simulink model "vehicle_model_controller"  (R2020b)
settings: Solver=VariableStepAuto  StartTime=0.0  StopTime=10.0  RelTol=1e-3
undefined symbols (not defined in the file or in its folder): BWLF, BWRF, front_forces, FWLF, FWRF, rear_forces
libraries: nesl_utility x24, sdl_lib x16, fl_lib x4, autolibmappedmotor x4, autolibdatasheetbattery x1, vehdynlibsteering x1, pid_lib x1, autolibshared x1
(part 1 of 2)
settings Model: Creator=True  LastModifiedBy=Inver
settings DataIOCC: ExternalInput=half_track_front.getElement(1),[],[],[],[],[],[],[],[],[],[]  LoadExternalInput=on
settings DebuggingCC: ArithmeticOperatorsInVariantConditions=warning
settings SFSimCC: CustomCodeUndefinedFunction=UseInterfaceOnly

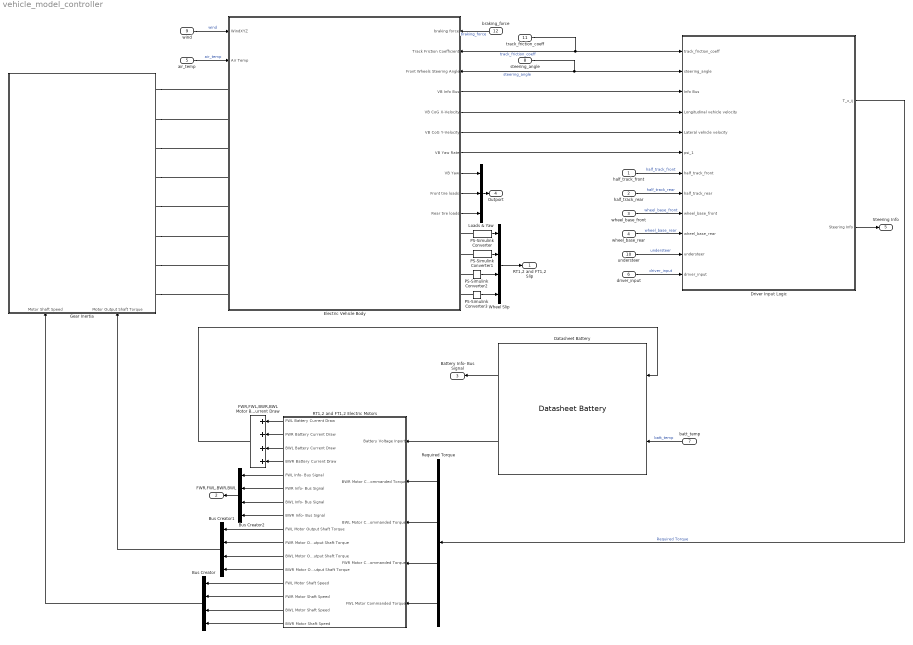
== system vehicle_model_controller ==
  half_track_front : Inport
  half_track_rear : Inport  Port=2
  wheel_base_front : Inport  Port=3
  wheel_base_rear : Inport  Port=4
  air_temp : Inport  Port=5
  driver_input : Inport  Port=6
  batt_temp : Inport  Port=7
  steering_angle : Inport  Port=8
  wind : Inport  Port=9
  understeer : Inport  Port=10
  track_friction_coeff : Inport  Port=11
  braking_force : Inport  Port=12
  Bus Creator : BusCreator  Inputs=FWL Speed,FWR Speed,BWL Speed,BWR Speed
  Bus Creator1 : BusCreator  Inputs=FWL Torque,FWR Torque,BWL Torque,BWR Torque
  Bus Creator2 : BusCreator  Inputs=4
  Datasheet Battery : autolibdatasheetbattery/Datasheet Battery  CapacityCtrl=Parameter  OutputVlt=Unfiltered  BattChargeMax=100  Em=[2.8 3.228 3.284 3.361 3.408 3.427 3.472 3.477 3.493 3.504 3.516 3.528 3.537 3.545 3.555 3.561 3.566 3.576 3.587 3.589 3.594 3.6 3.608 3.61 3.616 3.619 3.626 3.632 3.637 3.64 3.645 3.646 3.652 3.655 3.658 3.661 3.664 3.668 3.673 3.678 3.68 3.681 3.686 3.692 3.699 3.702 3.705 3.71 3.717 3.723 3.728 3.733 3.735 3.742 3.749 3.755 3.761 3.768 3.773 3.78 3.791 3.798 3.798 3.814 3.818 3.825 3.841 3.846 3.855 3.863 3.877 3.885 3.894 3.907 3.919 3.926 3.935 3.944 3.954 3.964 3.974 3.988 3.998 4.014 4.029 4.034 4.047 4.065 4.074 4.086 4.097 4.131 4.126 4.138 4.15 4.18 4.174 4.187 4.207 4.231 4.221]  CapLUTBp=[0 0.01 0.02 0.03 0.04 0.05 0.06 0.07 0.08 0.09 0.1 0.11 0.12 0.13 0.14 0.15 0.16 0.17 0.18 0.19 0.2 0.21 0.22 0.23 0.24 0.25 0.26 0.27 0.28 0.29 0.3 0.31 0.32 0.33 0.34 0.35 0.36 0.37 0.38 0.39 0.4 0.41 0.42 0.43 0.44 0.45 0.46 0.47 0.48 0.49 0.5 0.51 0.52 0.53 0.54 0.55 0.56 0.57 0.58 0.59 0.6 0.61 0.62 0.63 0.64 0.65 0.66 0.67 0.68 0.69 0.7 0.71 0.72 0.73 0.74 0.75 0.76 0.77 0.78 0.79 0.8 0.81 0.82 0.83 0.84 0.85 0.86 0.87 0.88 0.89 0.9 0.91 0.92 0.93 0.94 0.95 0.96 0.97 0.98 0.99 1]  RInt=[0.008846 0.009319 0.009027 0.00847 0.01032 0.01314;0.006389 0.006554 0.005553 0.005525 0.006043 0.007805;0.004364 0.004101 0.00406 0.003452 0.003846 0.004517;0.002031 0.002563 0.002532 0.00246 0.002716 0.003047;0.001443 0.001825 0.001795 0.001778 0.001924 0.002234;0.0005603 0.0007192 0.0006887 0.0007557 0.0007355 0.001014;0.001028 0.001338 0.001 0.001536 0.001546 0.002789]  BattTempBp=[243.1 253.1 263.1 273.1 283.1 298.1 313.1]  CapSOCBp=[0 0.2 0.4 0.6 0.8 1]  Ns=1  Np=1  BattCapInit=100  Tc=1/1000  Vinit=4.221  RefBlkName='autolibdatasheetbattery/Datasheet Battery'
      settings: SourceProductBaseCode=PW
  Driver Input Logic : Subsystem
  Electric Vehicle Body : Subsystem
      settings: PortSchema="{\"entries\":[{\"content\":{\"sides\":[{\"content\":{\"connectorIds\":[\"In1\",\"In2\",\"LConn1\",\"LConn2\",\"LConn3\",\"LConn4\",\"LConn5\",\"LConn6\",\"LConn7\",\"LConn8\"]},\"type\":\"ConnectorPlacement.EquallySpacedRectSide\",\"uuid\":\"d116468d-7868-487f-a964-21d40fbcc809\"},{\"content\":{\"connectorIds\":[\"In3\",\"In4\",\"In5\",\"Out1\",\"Out2\",\"Out3\",\"Out4\",\"Out5\",\"Out6\",\"Out7\",\"RConn1\",\"RConn2\",\"RConn3\",\"RConn4\"],\"side\":\"RIGHT\"},\"type\":\"ConnectorPlacement.EquallySpacedRectSide\",\"uuid\":\"69901164-3ba1-4787-94a1-b6dad3f5570f\"},{\"content\":{\"connectorIds\":[],\"side\":\"TOP\"},\"type\":\"ConnectorPlacement.EquallySpacedRectSide\",\"uuid\":\"0399aa14-7cbc-406a-a0bc-5234930aa618\"},{\"content\":{\"connectorIds\":[],\"side\":\"HIDDEN\"},\"type\":\"ConnectorPlacement.EquallySpacedRectSide\",\"uuid\":\"c7425876-ea80-44ac-a5c9-676a45313985\"}]},\"type\":\"ConnectorPlacement.EquallySpacedConnector\",\"uuid\":\"33585625-d9f5-41d4-8b4d-b29cb62e09b6\"}],\"packageUris\":[\"http://schema.mathworks.com/mf0/Connector/R2020b\"],\"version\":\"1.0\"}"
  FWR,FWL,BWR,BWL Motor Battery Current Draw : Sum  Inputs=++++
  Gear Inertia : Subsystem
      settings: PortSchema="{\"entries\":[{\"content\":{\"sides\":[{\"content\":{\"connectorIds\":[]},\"type\":\"ConnectorPlacement.EquallySpacedRectSide\",\"uuid\":\"d2da853d-f72f-405f-97f5-14de81bcd5cf\"},{\"content\":{\"connectorIds\":[\"RConn1\",\"RConn2\",\"RConn3\",\"RConn4\",\"RConn5\",\"RConn6\",\"RConn7\",\"RConn8\"],\"side\":\"RIGHT\"},\"type\":\"ConnectorPlacement.EquallySpacedRectSide\",\"uuid\":\"46df577e-3ff5-4d09-9a0c-c2313587257d\"},{\"content\":{\"connectorIds\":[],\"side\":\"TOP\"},\"type\":\"ConnectorPlacement.EquallySpacedRectSide\",\"uuid\":\"3ac7701d-a0be-47f8-b1ff-78174d996b09\"},{\"content\":{\"connectorIds\":[\"In1\",\"In2\"],\"side\":\"BOTTOM\"},\"type\":\"ConnectorPlacement.EquallySpacedRectSide\",\"uuid\":\"cde220f9-0c3d-4970-b228-0d476a2943e7\"},{\"content\":{\"connectorIds\":[],\"side\":\"HIDDEN\"},\"type\":\"ConnectorPlacement.EquallySpacedRectSide\",\"uuid\":\"76366aef-65a3-435b-b679-82e74c90300f\"}]},\"type\":\"ConnectorPlacement.EquallySpacedConnector\",\"uuid\":\"e97a27ad-84e2-4fc1-b928-f989677c188c\"}],\"packageUris\":[\"http://schema.mathworks.com/mf0/Connector/R2020b\"],\"version\":\"1.0\"}"
  Loads & Yaw : Mux  Inputs=3
  PS-Simulink Converter{,1..3} (4 alike) : nesl_utility/PS-Simulink Converter  PhysicalDomain=network_engine_domain  SubClassName=ps_output  LeftPortType=input  RightPortType=output  PseudoPeriodic=off  Frequencies=[]  Unit=inherit  AffineConversion=off
  RT1,2 and FT1,2 Electric Motors : Subsystem
  Required Torque : Demux
  Wheel Slip : Mux
  RT1,2 and FT1,2 Slip : Outport
  FWR,FWL,BWR,BWL : Outport  Port=2
  Battery Info- Bus Signal : Outport  Port=3
  Outport : Outport  Port=4
  Steering Info : Outport  Port=5
  wires:
  Datasheet Battery/2 -> RT1,2 and FT1,2 Electric Motors/1(Battery Voltage Inport)
  RT1,2 and FT1,2 Electric Motors/1(FWL Battery Current Draw) -> FWR,FWL,BWR,BWL Motor Battery Current Draw/1
  RT1,2 and FT1,2 Electric Motors/2(FWR Battery Current Draw) -> FWR,FWL,BWR,BWL Motor Battery Current Draw/2
  RT1,2 and FT1,2 Electric Motors/3(BWL Battery Current Draw) -> FWR,FWL,BWR,BWL Motor Battery Current Draw/3
  RT1,2 and FT1,2 Electric Motors/4(BWR Battery Current Draw) -> FWR,FWL,BWR,BWL Motor Battery Current Draw/4
  FWR,FWL,BWR,BWL Motor Battery Current Draw/1 -> Datasheet Battery/1
  PS-Simulink Converter/1 -> Wheel Slip/1
  PS-Simulink Converter1/1 -> Wheel Slip/2
  PS-Simulink Converter2/1 -> Wheel Slip/3
  PS-Simulink Converter3/1 -> Wheel Slip/4
  Wheel Slip/1 -> RT1,2 and FT1,2 Slip/1
  RT1,2 and FT1,2 Electric Motors/5(FWL Info- Bus Signal) -> Bus Creator2/1
  RT1,2 and FT1,2 Electric Motors/6(FWR Info- Bus Signal) -> Bus Creator2/2
  RT1,2 and FT1,2 Electric Motors/7(BWL Info- Bus Signal) -> Bus Creator2/3
  RT1,2 and FT1,2 Electric Motors/8(BWR Info- Bus Signal) -> Bus Creator2/4
  RT1,2 and FT1,2 Electric Motors/14(FWR Motor Shaft Speed) -> Bus Creator/2
  RT1,2 and FT1,2 Electric Motors/15(BWL Motor Shaft Speed) -> Bus Creator/3
  RT1,2 and FT1,2 Electric Motors/16(BWR Motor Shaft Speed) -> Bus Creator/4
  RT1,2 and FT1,2 Electric Motors/13(FWL Motor Shaft Speed) -> Bus Creator/1
  Datasheet Battery/1 -> Battery Info- Bus Signal/1
  RT1,2 and FT1,2 Electric Motors/9(FWL Motor Output Shaft Torque) -> Bus Creator1/1
  RT1,2 and FT1,2 Electric Motors/10(FWR Motor Output Shaft Torque) -> Bus Creator1/2
  RT1,2 and FT1,2 Electric Motors/11(BWL Motor Output Shaft Torque) -> Bus Creator1/3
  RT1,2 and FT1,2 Electric Motors/12(BWR Motor Output Shaft Torque) -> Bus Creator1/4
  Required Torque/4 -> RT1,2 and FT1,2 Electric Motors/5(FWL Motor Commanded Torque)
  Required Torque/3 -> RT1,2 and FT1,2 Electric Motors/4("FWR Motor Commanded Torque ")
  Required Torque/2 -> RT1,2 and FT1,2 Electric Motors/3(BWL Motor Commanded Torque)
  Required Torque/1 -> RT1,2 and FT1,2 Electric Motors/2(BWR Motor Commanded Torque)
  Loads & Yaw/1 -> Outport/1
  Electric Vehicle Body/5(VB Yaw) -> Loads & Yaw/1
  Electric Vehicle Body/6(Front tire loads) -> Loads & Yaw/2
  Electric Vehicle Body/7(Rear tire loads) -> Loads & Yaw/3
  Bus Creator2/1 -> FWR,FWL,BWR,BWL/1
  Bus Creator1/1 -> Gear Inertia/2(Motor Output Shaft Torque)
  Bus Creator/1 -> Gear Inertia/1(Motor Shaft Speed)
  air_temp/1 -> Electric Vehicle Body/2(Air Temp)  "air_temp"
  wind/1 -> Electric Vehicle Body/1(WindXYZ)  "wind"
  batt_temp/1 -> Datasheet Battery/2  "batt_temp"
  track_friction_coeff/1 -> Driver Input Logic/1(track_friction_coeff), Electric Vehicle Body/4(Track Friction Coefficient)  "track_friction_coeff"
  steering_angle/1 -> Electric Vehicle Body/5(Front Wheels Steering Angle), Driver Input Logic/2(steering_angle)  "steering_angle"
  Electric Vehicle Body/1(VB Info Bus) -> Driver Input Logic/3(Info Bus)
  Electric Vehicle Body/2("VB CoG X-Velocity ") -> Driver Input Logic/4(Longitudinal vehicle velocity)
  Electric Vehicle Body/3(VB CoG Y-Velocity) -> Driver Input Logic/5(Lateral vehicle velocity)
  Electric Vehicle Body/4(VB Yaw Rate) -> Driver Input Logic/6(psi_1)
  half_track_front/1 -> Driver Input Logic/7(half_track_front)  "half_track_front"
  half_track_rear/1 -> Driver Input Logic/8(half_track_rear)  "half_track_rear"
  wheel_base_front/1 -> Driver Input Logic/9(wheel_base_front)  "wheel_base_front"
  wheel_base_rear/1 -> Driver Input Logic/10(wheel_base_rear)  "wheel_base_rear"
  understeer/1 -> Driver Input Logic/11(understeer)  "understeer"
  driver_input/1 -> Driver Input Logic/12(driver_input)  "driver_input"
  Driver Input Logic/1(T_x_ij) -> Required Torque/1  "Required Torque"
  Driver Input Logic/2(Steering Info) -> Steering Info/1
  braking_force/1 -> Electric Vehicle Body/3(braking force)  "braking_force"
  connections:
  PS-Simulink Converter/LConn1 -- Electric Vehicle Body/RConn1
  PS-Simulink Converter1/LConn1 -- Electric Vehicle Body/RConn2
  PS-Simulink Converter2/LConn1 -- Electric Vehicle Body/RConn3
  PS-Simulink Converter3/LConn1 -- Electric Vehicle Body/RConn4
  Gear Inertia/RConn1 -- Electric Vehicle Body/LConn1
  Gear Inertia/RConn2 -- Electric Vehicle Body/LConn2
  Gear Inertia/RConn3 -- Electric Vehicle Body/LConn3
  Gear Inertia/RConn4 -- Electric Vehicle Body/LConn4
  Gear Inertia/RConn5 -- Electric Vehicle Body/LConn5
  Gear Inertia/RConn6 -- Electric Vehicle Body/LConn6
  Gear Inertia/RConn7 -- Electric Vehicle Body/LConn7
  Gear Inertia/RConn8 -- Electric Vehicle Body/LConn8

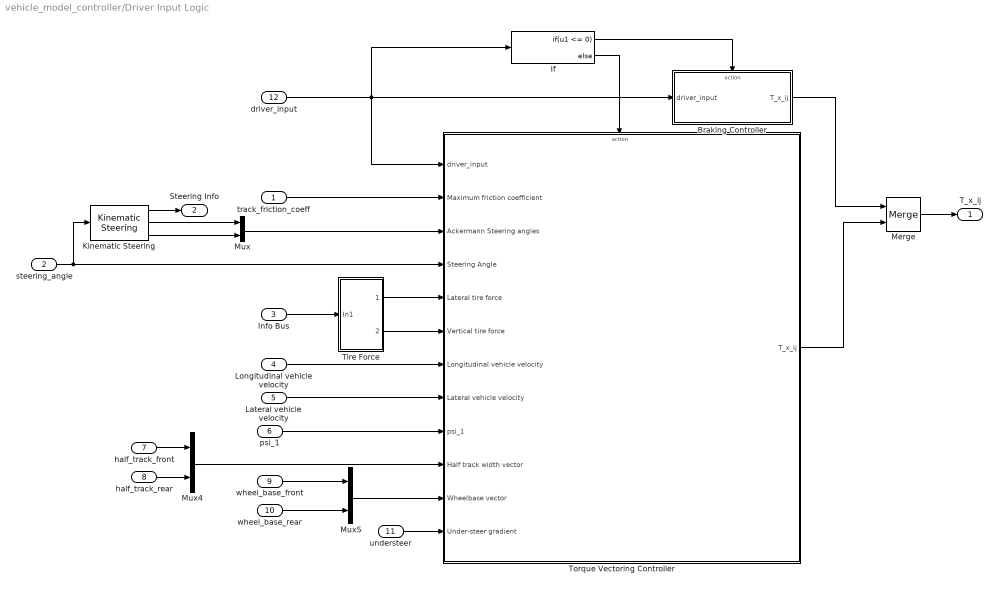
== system vehicle_model_controller/Driver Input Logic ==
  track_friction_coeff : Inport
  steering_angle : Inport  Port=2
  Info Bus : Inport  Port=3
  Longitudinal vehicle velocity : Inport  Port=4
  Lateral vehicle velocity : Inport  Port=5
  psi_1 : Inport  Port=6
  half_track_front : Inport  Port=7
  half_track_rear : Inport  Port=8
  wheel_base_front : Inport  Port=9
  wheel_base_rear : Inport  Port=10
  understeer : Inport  Port=11
  driver_input : Inport  Port=12
  Braking Controller : Subsystem
  If : If  IfExpression=u1 <= 0
  Kinematic Steering : vehdynlibsteering/Kinematic Steering  StrgType=Ackerman  StrgRatioType=Constant  Loc=Front  NrmlFctr=0.01  TrckWdth=1  WhlBase=1.524  Db=0  StrgRng=1.25*pi  StrgAngBpts="[-6.2832   -5.0265   -3.7699   -2.5133   -1.2566         0    1.2566    2.5133    3.7699    5.0265    6.2832]"  StrgRatioTbl=|  StrgRatio=100  StrgArmLngth=0.1  RckCsLngth=0.5  TieRodLngth=0.248  D=0.2  PnnRadius=0.0057  PnnRadiusTbl="[0.0055    0.0055    0.0056    0.0057    0.0058    0.0057    0.0057    0.0057    0.0056    0.0055    0.0055]"  RodLngth=0.1  ParaArmLngth=0.9  aMode=2
      | [13.5000   13.3750   13.2500   13.1250   13.0000   13.0000   13.0000   13.1250   13.2500   13.3750   13.5000
      | ]
  Merge : Merge
  Mux : Mux  Inputs=2
  Mux4 : Mux  Inputs=2
  Mux5 : Mux  Inputs=2
  Tire Force : Subsystem
  Torque Vectoring Controller : Subsystem
  T_x_ij : Outport
  Steering Info : Outport  Port=2
  wires:
  Mux4/1 -> Torque Vectoring Controller/10(Half track width vector)
  understeer/1 -> Torque Vectoring Controller/12(Under-steer gradient)
  Tire Force/1(Lateral) -> Torque Vectoring Controller/5(Lateral tire force)
  Lateral vehicle velocity/1 -> Torque Vectoring Controller/8(Lateral vehicle velocity)
  Mux5/1 -> Torque Vectoring Controller/11(Wheelbase vector)
  Longitudinal vehicle velocity/1 -> Torque Vectoring Controller/7(Longitudinal vehicle velocity)
  Tire Force/2(Vertical) -> Torque Vectoring Controller/6(Vertical tire force)
  Info Bus/1 -> Tire Force/1(In1)
  half_track_front/1 -> Mux4/1
  half_track_rear/1 -> Mux4/2
  wheel_base_rear/1 -> Mux5/2
  wheel_base_front/1 -> Mux5/1
  psi_1/1 -> Torque Vectoring Controller/9(psi_1)
  track_friction_coeff/1 -> Torque Vectoring Controller/2(Maximum friction coefficient)
  If/1 -> Braking Controller/Action
  Merge/1 -> T_x_ij/1
  If/2 -> Torque Vectoring Controller/Action
  Braking Controller/1(T_x_ij) -> Merge/1
  Torque Vectoring Controller/1(T_x_ij) -> Merge/2
  driver_input/1 -> Braking Controller/1(driver_input), Torque Vectoring Controller/1(driver_input), If/1
  Kinematic Steering/3 -> Mux/2
  Kinematic Steering/2 -> Mux/1
  steering_angle/1 -> Torque Vectoring Controller/4(Steering Angle), Kinematic Steering/1
  Mux/1 -> Torque Vectoring Controller/3("Ackermann Steering angles ")
  Kinematic Steering/1 -> Steering Info/1

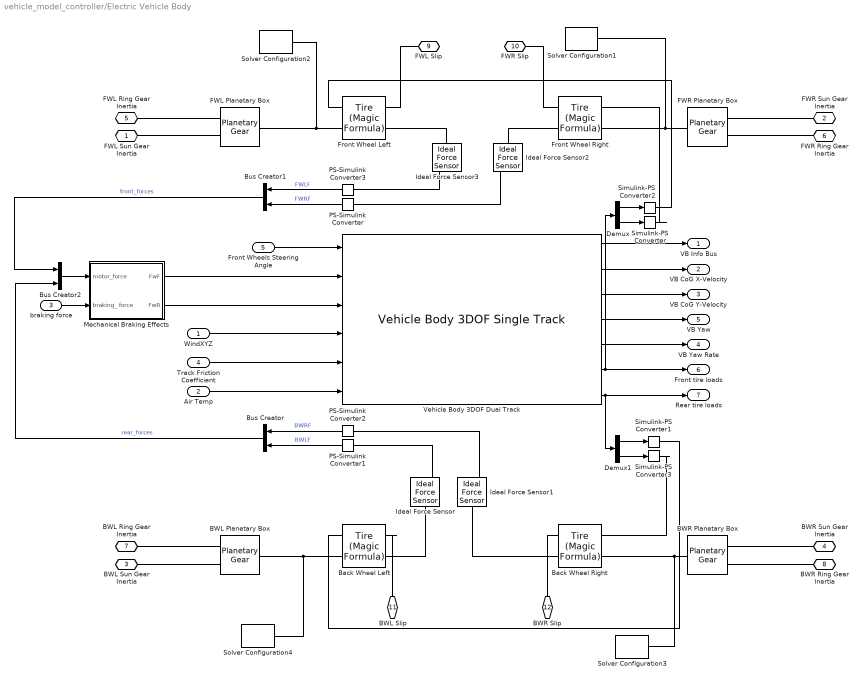
== system vehicle_model_controller/Electric Vehicle Body ==
  WindXYZ : Inport
  Air Temp : Inport  Port=2
  braking force : Inport  Port=3
  Track Friction Coefficient : Inport  Port=4
  Front Wheels Steering Angle : Inport  Port=5
  BWL Planetary Box : sdl_lib/Gears/Planetary Gear  rs_ratio=2  friction_model=sdl.enum.gear_friction.none  mu_visc=[0, 0] N*m/(rad/s)  efficiency=[.96, .98]  temperature_TLU=[280, 300, 320] K  efficiency_sp_TLU=[.95, .9, .85]  efficiency_rp_TLU=[.95, .9, .85]  pwr_thr=[.001, .001] W  thermal_mass=50 J/K  T_init=300 K  model_inertia=simscape.enum.onoff.off  planet_inertia=0.001 kg*m^2
      settings: SourceProductBaseCode=LD
  BWR Planetary Box : sdl_lib/Gears/Planetary Gear  rs_ratio=2  friction_model=sdl.enum.gear_friction.none  mu_visc=[0, 0] N*m/(rad/s)  efficiency=[.96, .98]  temperature_TLU=[280, 300, 320] K  efficiency_sp_TLU=[.95, .9, .85]  efficiency_rp_TLU=[.95, .9, .85]  pwr_thr=[.001, .001] W  thermal_mass=50 J/K  T_init=300 K  model_inertia=simscape.enum.onoff.off  planet_inertia=0.001 kg*m^2
      settings: SourceProductBaseCode=LD
  Back Wheel Left : sdl_lib/Tires & Vehicles/Tire (Magic Formula)  parameterization=sdl.enum.magic_tire_model.peak  F_z1=3000 N  F_x1=3500 N  kappa1=10  B_m=10  C_m=1.9  D_m=1  E_m=0.97  fz0=4000 N  p_Cx=1.685  p_Dx=[1.21, -.037]  p_Ex=[.344, .095, -.02, 0]  p_Kx=[21.51, -.163, .245]  p_Hx=[-.002, .002]  p_Vx=[0, 0]  v_tr_thr=0.1 m/s  r_e=0.3 m  model_compliance=0  stiffness=1e6 N/m  damping=1000 N/(m/s)  model_inertia=0  inertia=1 kg*m^2  initial_velocity=0 rad/s  model_resistance=0  resistance_model=1  coeff=0.015  p_tire=250e3 Pa  alpha=-0.003  beta=0.97  coeff_a=84e-4  coeff_b=6.2e-4 s/m  coeff_c=1.6e-4 s^2/m^2  v_thr=0.001 m/s
  Back Wheel Right : sdl_lib/Tires & Vehicles/Tire (Magic Formula)  parameterization=sdl.enum.magic_tire_model.peak  F_z1=3000 N  F_x1=3500 N  kappa1=10  B_m=10  C_m=1.9  D_m=1  E_m=0.97  fz0=4000 N  p_Cx=1.685  p_Dx=[1.21, -.037]  p_Ex=[.344, .095, -.02, 0]  p_Kx=[21.51, -.163, .245]  p_Hx=[-.002, .002]  p_Vx=[0, 0]  v_tr_thr=0.1 m/s  r_e=0.3 m  model_compliance=0  stiffness=1e6 N/m  damping=1000 N/(m/s)  model_inertia=0  inertia=1 kg*m^2  initial_velocity=0 rad/s  model_resistance=0  resistance_model=1  coeff=0.015  p_tire=250e3 Pa  alpha=-0.003  beta=0.97  coeff_a=84e-4  coeff_b=6.2e-4 s/m  coeff_c=1.6e-4 s^2/m^2  v_thr=0.001 m/s
  Bus Creator : BusCreator  Inputs=BWRF,BWLF
  Bus Creator1 : BusCreator  Inputs=FWLF,FWRF
  Bus Creator2 : BusCreator  Inputs=front_forces,rear_forces
  Demux : Demux  Outputs=2
  Demux1 : Demux  Outputs=2
  FWL Planetary Box : sdl_lib/Gears/Planetary Gear  rs_ratio=2  friction_model=sdl.enum.gear_friction.none  mu_visc=[0, 0] N*m/(rad/s)  efficiency=[.96, .98]  temperature_TLU=[280, 300, 320] K  efficiency_sp_TLU=[.95, .9, .85]  efficiency_rp_TLU=[.95, .9, .85]  pwr_thr=[.001, .001] W  thermal_mass=50 J/K  T_init=300 K  model_inertia=simscape.enum.onoff.off  planet_inertia=0.001 kg*m^2
      settings: SourceProductBaseCode=LD
  FWR Planetary Box : sdl_lib/Gears/Planetary Gear  rs_ratio=2  friction_model=sdl.enum.gear_friction.none  mu_visc=[0, 0] N*m/(rad/s)  efficiency=[.96, .98]  temperature_TLU=[280, 300, 320] K  efficiency_sp_TLU=[.95, .9, .85]  efficiency_rp_TLU=[.95, .9, .85]  pwr_thr=[.001, .001] W  thermal_mass=50 J/K  T_init=300 K  model_inertia=simscape.enum.onoff.off  planet_inertia=0.001 kg*m^2
      settings: SourceProductBaseCode=LD
  Front Wheel Left : sdl_lib/Tires & Vehicles/Tire (Magic Formula)  parameterization=sdl.enum.magic_tire_model.peak  F_z1=3000 N  F_x1=3500 N  kappa1=10  B_m=10  C_m=1.9  D_m=1  E_m=0.97  fz0=4000 N  p_Cx=1.685  p_Dx=[1.21, -.037]  p_Ex=[.344, .095, -.02, 0]  p_Kx=[21.51, -.163, .245]  p_Hx=[-.002, .002]  p_Vx=[0, 0]  v_tr_thr=0.1 m/s  r_e=0.3 m  model_compliance=0  stiffness=1e6 N/m  damping=1000 N/(m/s)  model_inertia=0  inertia=1 kg*m^2  initial_velocity=0 rad/s  model_resistance=0  resistance_model=1  coeff=0.015  p_tire=250e3 Pa  alpha=-0.003  beta=0.97  coeff_a=84e-4  coeff_b=6.2e-4 s/m  coeff_c=1.6e-4 s^2/m^2  v_thr=0.001 m/s
  Front Wheel Right : sdl_lib/Tires & Vehicles/Tire (Magic Formula)  parameterization=sdl.enum.magic_tire_model.peak  F_z1=3000 N  F_x1=3500 N  kappa1=10  B_m=10  C_m=1.9  D_m=1  E_m=0.97  fz0=4000 N  p_Cx=1.685  p_Dx=[1.21, -.037]  p_Ex=[.344, .095, -.02, 0]  p_Kx=[21.51, -.163, .245]  p_Hx=[-.002, .002]  p_Vx=[0, 0]  v_tr_thr=0.1 m/s  r_e=0.3 m  model_compliance=0  stiffness=1e6 N/m  damping=1000 N/(m/s)  model_inertia=0  inertia=1 kg*m^2  initial_velocity=0 rad/s  model_resistance=0  resistance_model=1  coeff=0.015  p_tire=250e3 Pa  alpha=-0.003  beta=0.97  coeff_a=84e-4  coeff_b=6.2e-4 s/m  coeff_c=1.6e-4 s^2/m^2  v_thr=0.001 m/s
  Ideal Force Sensor{,1..3} (4 alike) : fl_lib/Mechanical/Mechanical Sensors/Ideal Force Sensor
  Mechanical Braking Effects : Subsystem
  PS-Simulink Converter{,1..3} (4 alike) : nesl_utility/PS-Simulink Converter  PhysicalDomain=network_engine_domain  SubClassName=ps_output  LeftPortType=input  RightPortType=output  PseudoPeriodic=off  Frequencies=[]  Unit=inherit  AffineConversion=off
  Simulink-PS Converter{,1..3} (4 alike) : nesl_utility/Simulink-PS Converter  PhysicalDomain=network_engine_domain  SubClassName=ps_input  LeftPortType=input  RightPortType=output  PseudoPeriodic=off  Frequencies=[]  NoiseDistribution=none  NoiseParameters=[]  Unit=N  AffineConversion=off  FilteringAndDerivatives=provide  SimscapeFilterOrder=1  InputFilterTimeConstant=0.001  UdotUserProvided=0
  Solver Configuration{1..4} (4 alike) : nesl_utility/Solver Configuration  PhysicalDomain=network_engine_domain  SubClassName=solver  LeftPortType=input  RightPortType=generic  Tones=[]  Harmonics=[]  SimulateNoise=off  Profile=off  UseLocalSampling=off  EnableSwitchedLinearOptims=on  FrequencyDomain=off  UseCCode=off  RelTol=0.001  AbsTol=1e-06  MinStep=1e-09  ToWorkspace=off  RevertToSquareIcSolve=off  NumHomotopyIterations=100  PhasorMode=off  PhasorModeNumHarmonics=1  DoDC=off  ResidualTolerance=1e-09  UseLocalSolver=off  LocalSolverChoice=NE_BACKWARD_EULER_ADVANCER  LocalSolverSampleTime=0.001  DoFixedCost=off  MaxNonlinIter=3  MaxModeIter=2  ComputeImpulses=off  ImpulseIterations=2  LinearAlgebra=auto  EquationFormulation=NE_TIME_EF  DelaysMemoryBudget=1024  AutomaticFiltering=on  FilteringTimeConstant=0.001  PartitionStorageMethod=AS_NEEDED  PartitionMemoryBudget=1024  PartitionMethod=ROBUST
  Vehicle Body 3DOF Dual Track : autolibshared/Vehicle Body 3DOF Single Track  trackMode=Dual  inputMode=External longitudinal forces  frontSteerMode=on  rearSteerMode=off  windMode=on  muMode=on  extFMode=off  extMMode=off  htchFMode=off  htchMMode=off  extXo=off  extpsio=off  extxdoto=off  extro=off  extYo=off  extTamb=on  extydoto=off  aMode=2  NF=2  NR=2  m=223  a=1.5  b=1.5  h=0.35  dh=1  hh=0.2  X_o=0  xdot_o=0  CalphaMode=off  sigmaMode=on  d=0  hl=0  w=[1.4,1.4]  Cy_f=12e3  Cy_r=11e3  sigma_f=.1  sigma_r=.1  alpha_f_brk=[-.1 .1]  Cy_f_data=[-9e3 9e3]  alpha_r_brk=[-.1 .1]  Cy_r_data=[-9e3 9e3]  Y_o=0  ydot_o=0  Izz=4000  psi_o=0  r_o=0  Af=2  Cd=.3  Cl=.1  Cpm=.1  beta_w=[0:0.01:0.3]  Cs=[0:0.03:0.9]  Cym=[0:0.01:0.3]  Pabs=101325  Tair=273  g=9.81  mu=1  xdot_tol=.01  Fznom=5000  Fxtire_sat=7e4  Fytire_sat=7e4  longOff=0  latOff=0  vertOff=0  wrapAng=off
      settings: SourceProductBaseCode=PW,MT,UV,VE,VP
  FWL Sun Gear Inertia : PMIOPort  Side=Left
  FWR Sun Gear Inertia : PMIOPort  Port=2  Side=Left
  BWL Sun Gear Inertia : PMIOPort  Port=3  Side=Left
  BWR Sun Gear Inertia : PMIOPort  Port=4  Side=Left
  FWL Ring Gear Inertia : PMIOPort  Port=5  Side=Left
  FWR Ring Gear Inertia : PMIOPort  Port=6  Side=Left
  BWL Ring Gear Inertia : PMIOPort  Port=7  Side=Left
  BWR Ring Gear Inertia : PMIOPort  Port=8  Side=Left
  FWL Slip : PMIOPort  Port=9  Side=Right
  FWR Slip : PMIOPort  Port=10  Side=Right
  BWL Slip : PMIOPort  Port=11  Side=Right
  BWR Slip : PMIOPort  Port=12  Side=Right
  VB Info Bus : Outport
  "VB CoG X-Velocity " : Outport  Port=2
  VB CoG Y-Velocity : Outport  Port=3
  VB Yaw Rate : Outport  Port=4
  VB Yaw : Outport  Port=5
  Front tire loads : Outport  Port=6
  Rear tire loads : Outport  Port=7
  wires:
  Vehicle Body 3DOF Dual Track/6 -> Front tire loads/1, Demux/1
  Vehicle Body 3DOF Dual Track/7 -> Rear tire loads/1, Demux1/1
  Air Temp/1 -> Vehicle Body 3DOF Dual Track/6
  Front Wheels Steering Angle/1 -> Vehicle Body 3DOF Dual Track/1
  Track Friction Coefficient/1 -> Vehicle Body 3DOF Dual Track/5
  WindXYZ/1 -> Vehicle Body 3DOF Dual Track/4
  Vehicle Body 3DOF Dual Track/1 -> VB Info Bus/1
  Vehicle Body 3DOF Dual Track/2 -> "VB CoG X-Velocity "/1
  Vehicle Body 3DOF Dual Track/3 -> VB CoG Y-Velocity/1
  Vehicle Body 3DOF Dual Track/4 -> VB Yaw/1
  Vehicle Body 3DOF Dual Track/5 -> VB Yaw Rate/1
  Mechanical Braking Effects/2(FwR) -> Vehicle Body 3DOF Dual Track/3
  Mechanical Braking Effects/1(FwF) -> Vehicle Body 3DOF Dual Track/2
  Demux/2 -> Simulink-PS Converter/1
  Demux/1 -> Simulink-PS Converter2/1
  Demux1/1 -> Simulink-PS Converter1/1
  Demux1/2 -> Simulink-PS Converter3/1
  PS-Simulink Converter2/1 -> Bus Creator/1  "BWRF"
  PS-Simulink Converter1/1 -> Bus Creator/2  "BWLF"
  PS-Simulink Converter3/1 -> Bus Creator1/1  "FWLF"
  PS-Simulink Converter/1 -> Bus Creator1/2  "FWRF"
  Bus Creator/1 -> Bus Creator2/2  "rear_forces"
  braking force/1 -> Mechanical Braking Effects/2(braking_	force)
  Bus Creator1/1 -> Bus Creator2/1  "front_forces"
  Bus Creator2/1 -> Mechanical Braking Effects/1(motor_force)
  connections:
  Ideal Force Sensor/LConn1 -- Back Wheel Left/RConn2
  FWL Ring Gear Inertia/RConn1 -- FWL Planetary Box/RConn1
  BWR Ring Gear Inertia/RConn1 -- BWR Planetary Box/RConn1
  BWL Ring Gear Inertia/RConn1 -- BWL Planetary Box/RConn1
  Back Wheel Left/LConn2 -- Solver Configuration4/RConn1 -- BWL Planetary Box/LConn1
  BWR Sun Gear Inertia/RConn1 -- BWR Planetary Box/RConn2
  Back Wheel Left/RConn1 -- BWL Slip/RConn1
  Front Wheel Right/RConn1 -- FWR Slip/RConn1
  BWL Sun Gear Inertia/RConn1 -- BWL Planetary Box/RConn2
  Front Wheel Left/RConn1 -- FWL Slip/RConn1
  FWR Ring Gear Inertia/RConn1 -- FWR Planetary Box/RConn1
  Back Wheel Right/RConn1 -- BWR Slip/RConn1
  FWR Planetary Box/LConn1 -- Solver Configuration1/RConn1 -- Front Wheel Right/LConn2
  Back Wheel Right/LConn2 -- Solver Configuration3/RConn1 -- BWR Planetary Box/LConn1
  FWL Sun Gear Inertia/RConn1 -- FWL Planetary Box/RConn2
  FWL Planetary Box/LConn1 -- Solver Configuration2/RConn1 -- Front Wheel Left/LConn2
  FWR Sun Gear Inertia/RConn1 -- FWR Planetary Box/RConn2
  PS-Simulink Converter/LConn1 -- Ideal Force Sensor2/RConn2
  Ideal Force Sensor/RConn2 -- PS-Simulink Converter1/LConn1
  Ideal Force Sensor1/LConn1 -- Back Wheel Right/RConn2
  Ideal Force Sensor1/RConn2 -- PS-Simulink Converter2/LConn1
  Ideal Force Sensor3/LConn1 -- Front Wheel Left/RConn2
  Ideal Force Sensor2/LConn1 -- Front Wheel Right/RConn2
  Ideal Force Sensor3/RConn2 -- PS-Simulink Converter3/LConn1
  Simulink-PS Converter2/RConn1 -- Front Wheel Left/LConn1
  Simulink-PS Converter/RConn1 -- Front Wheel Right/LConn1
  Simulink-PS Converter1/RConn1 -- Back Wheel Left/LConn1
  Simulink-PS Converter3/RConn1 -- Back Wheel Right/LConn1

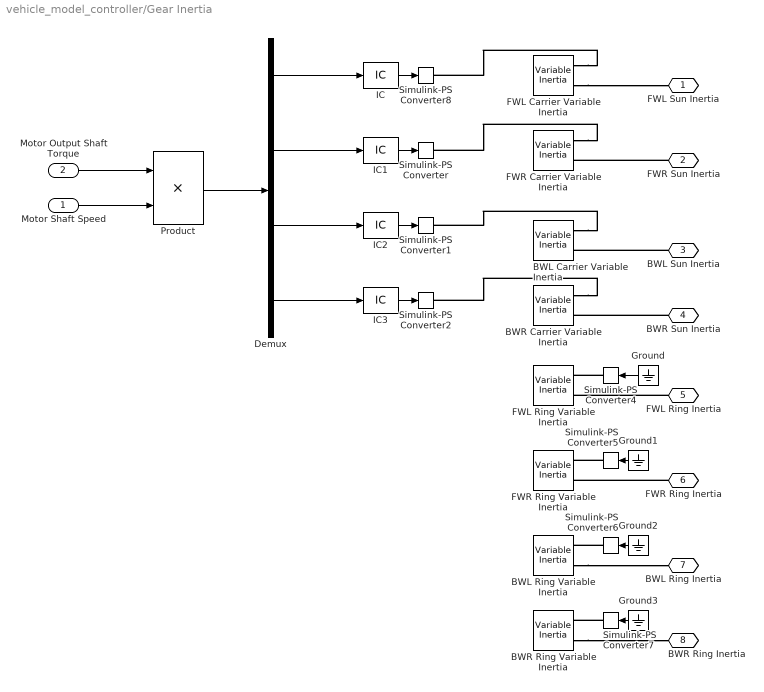
== system vehicle_model_controller/Gear Inertia ==
  Motor Shaft Speed : Inport
  Motor Output Shaft Torque : Inport  Port=2
  BWL Carrier Variable Inertia : sdl_lib/Inertias & Loads/Variable Inertia  minimum_inertia=0.1 kg*m^2  L_specify=off  L_priority=High  L=0 m^2*kg/s  L_nominal_specify=off  L_nominal_unit=m^2*kg/s  L_nominal_value=1
      settings: SourceProductBaseCode=LD  InternalSimscapePortConfiguration="{\"Bottom\":[],\"Left\":[{\"id\":\"I\",\"label\":\"\",\"type\":\"input\"},{\"id\":\"A\",\"label\":\"\",\"type\":\"foundation.mechanical.rotational.rotational\"}],\"Right\":[],\"Top\":[]}"
  BWL Ring Variable Inertia : sdl_lib/Inertias & Loads/Variable Inertia  minimum_inertia=0.1 kg*m^2  L_specify=off  L_priority=High  L=0 m^2*kg/s  L_nominal_specify=off  L_nominal_unit=m^2*kg/s  L_nominal_value=1
      settings: SourceProductBaseCode=LD  InternalSimscapePortConfiguration="{\"Bottom\":[],\"Left\":[{\"id\":\"I\",\"label\":\"\",\"type\":\"input\"},{\"id\":\"A\",\"label\":\"\",\"type\":\"foundation.mechanical.rotational.rotational\"}],\"Right\":[],\"Top\":[]}"
  BWR Carrier Variable Inertia : sdl_lib/Inertias & Loads/Variable Inertia  minimum_inertia=0.1 kg*m^2  L_specify=off  L_priority=High  L=0 m^2*kg/s  L_nominal_specify=off  L_nominal_unit=m^2*kg/s  L_nominal_value=1
      settings: SourceProductBaseCode=LD  InternalSimscapePortConfiguration="{\"Bottom\":[],\"Left\":[{\"id\":\"I\",\"label\":\"\",\"type\":\"input\"},{\"id\":\"A\",\"label\":\"\",\"type\":\"foundation.mechanical.rotational.rotational\"}],\"Right\":[],\"Top\":[]}"
  BWR Ring Variable Inertia : sdl_lib/Inertias & Loads/Variable Inertia  minimum_inertia=0.1 kg*m^2  L_specify=off  L_priority=High  L=0 m^2*kg/s  L_nominal_specify=off  L_nominal_unit=m^2*kg/s  L_nominal_value=1
      settings: SourceProductBaseCode=LD  InternalSimscapePortConfiguration="{\"Bottom\":[],\"Left\":[{\"id\":\"I\",\"label\":\"\",\"type\":\"input\"},{\"id\":\"A\",\"label\":\"\",\"type\":\"foundation.mechanical.rotational.rotational\"}],\"Right\":[],\"Top\":[]}"
  Demux : Demux
  FWL Carrier Variable Inertia : sdl_lib/Inertias & Loads/Variable Inertia  minimum_inertia=0.1 kg*m^2  L_specify=off  L_priority=High  L=0 m^2*kg/s  L_nominal_specify=off  L_nominal_unit=m^2*kg/s  L_nominal_value=1
      settings: SourceProductBaseCode=LD  InternalSimscapePortConfiguration="{\"Bottom\":[],\"Left\":[{\"id\":\"I\",\"label\":\"\",\"type\":\"input\"},{\"id\":\"A\",\"label\":\"\",\"type\":\"foundation.mechanical.rotational.rotational\"}],\"Right\":[],\"Top\":[]}"
  FWL Ring Variable Inertia : sdl_lib/Inertias & Loads/Variable Inertia  minimum_inertia=0.1 kg*m^2  L_specify=off  L_priority=High  L=0 m^2*kg/s  L_nominal_specify=off  L_nominal_unit=m^2*kg/s  L_nominal_value=1
      settings: SourceProductBaseCode=LD  InternalSimscapePortConfiguration="{\"Bottom\":[],\"Left\":[{\"id\":\"I\",\"label\":\"\",\"type\":\"input\"},{\"id\":\"A\",\"label\":\"\",\"type\":\"foundation.mechanical.rotational.rotational\"}],\"Right\":[],\"Top\":[]}"
  FWR Carrier Variable Inertia : sdl_lib/Inertias & Loads/Variable Inertia  minimum_inertia=0.1 kg*m^2  L_specify=off  L_priority=High  L=0 m^2*kg/s  L_nominal_specify=off  L_nominal_unit=m^2*kg/s  L_nominal_value=1
      settings: SourceProductBaseCode=LD  InternalSimscapePortConfiguration="{\"Bottom\":[],\"Left\":[{\"id\":\"I\",\"label\":\"\",\"type\":\"input\"},{\"id\":\"A\",\"label\":\"\",\"type\":\"foundation.mechanical.rotational.rotational\"}],\"Right\":[],\"Top\":[]}"
  FWR Ring Variable Inertia : sdl_lib/Inertias & Loads/Variable Inertia  minimum_inertia=0.1 kg*m^2  L_specify=off  L_priority=High  L=0 m^2*kg/s  L_nominal_specify=off  L_nominal_unit=m^2*kg/s  L_nominal_value=1
      settings: SourceProductBaseCode=LD  InternalSimscapePortConfiguration="{\"Bottom\":[],\"Left\":[{\"id\":\"I\",\"label\":\"\",\"type\":\"input\"},{\"id\":\"A\",\"label\":\"\",\"type\":\"foundation.mechanical.rotational.rotational\"}],\"Right\":[],\"Top\":[]}"
  Ground{,1..3} (4 alike) : Ground
  IC{,1..3} (4 alike) : InitialCondition  Value=0
  Product : Product
  Simulink-PS Converter{,1..2,4..8} (8 alike) : nesl_utility/Simulink-PS Converter  PhysicalDomain=network_engine_domain  SubClassName=ps_input  LeftPortType=input  RightPortType=output  PseudoPeriodic=off  Frequencies=[]  NoiseDistribution=none  NoiseParameters=[]  Unit=1  AffineConversion=off  FilteringAndDerivatives=provide  SimscapeFilterOrder=1  InputFilterTimeConstant=0.001  UdotUserProvided=0
  FWL Sun Inertia : PMIOPort  Side=Right
  FWR Sun Inertia : PMIOPort  Port=2  Side=Right
  BWL Sun Inertia : PMIOPort  Port=3  Side=Right
  BWR Sun Inertia : PMIOPort  Port=4  Side=Right
  FWL Ring Inertia : PMIOPort  Port=5  Side=Right
  FWR Ring Inertia : PMIOPort  Port=6  Side=Right
  BWL Ring Inertia : PMIOPort  Port=7  Side=Right
  BWR Ring Inertia : PMIOPort  Port=8  Side=Right
  wires:
  Ground1/1 -> Simulink-PS Converter5/1
  Ground2/1 -> Simulink-PS Converter6/1
  Ground3/1 -> Simulink-PS Converter7/1
  Ground/1 -> Simulink-PS Converter4/1
  Motor Output Shaft Torque/1 -> Product/1
  Motor Shaft Speed/1 -> Product/2
  Demux/1 -> IC/1
  Demux/2 -> IC1/1
  Demux/3 -> IC2/1
  Demux/4 -> IC3/1
  IC/1 -> Simulink-PS Converter8/1
  IC1/1 -> Simulink-PS Converter/1
  IC2/1 -> Simulink-PS Converter1/1
  IC3/1 -> Simulink-PS Converter2/1
  Product/1 -> Demux/1
  connections:
  BWR Carrier Variable Inertia/LConn1 -- Simulink-PS Converter2/RConn1
  BWL Sun Inertia/RConn1 -- BWL Carrier Variable Inertia/LConn2
  FWL Carrier Variable Inertia/LConn1 -- Simulink-PS Converter8/RConn1
  BWL Carrier Variable Inertia/LConn1 -- Simulink-PS Converter1/RConn1
  FWR Sun Inertia/RConn1 -- FWR Carrier Variable Inertia/LConn2
  FWL Carrier Variable Inertia/LConn2 -- FWL Sun Inertia/RConn1
  FWR Carrier Variable Inertia/LConn1 -- Simulink-PS Converter/RConn1
  BWR Sun Inertia/RConn1 -- BWR Carrier Variable Inertia/LConn2
  BWL Ring Variable Inertia/LConn2 -- BWL Ring Inertia/RConn1
  Simulink-PS Converter6/RConn1 -- BWL Ring Variable Inertia/LConn1
  FWR Ring Inertia/RConn1 -- FWR Ring Variable Inertia/LConn2
  Simulink-PS Converter5/RConn1 -- FWR Ring Variable Inertia/LConn1
  BWR Ring Variable Inertia/LConn2 -- BWR Ring Inertia/RConn1
  Simulink-PS Converter7/RConn1 -- BWR Ring Variable Inertia/LConn1
  Simulink-PS Converter4/RConn1 -- FWL Ring Variable Inertia/LConn1
  FWL Ring Inertia/RConn1 -- FWL Ring Variable Inertia/LConn2

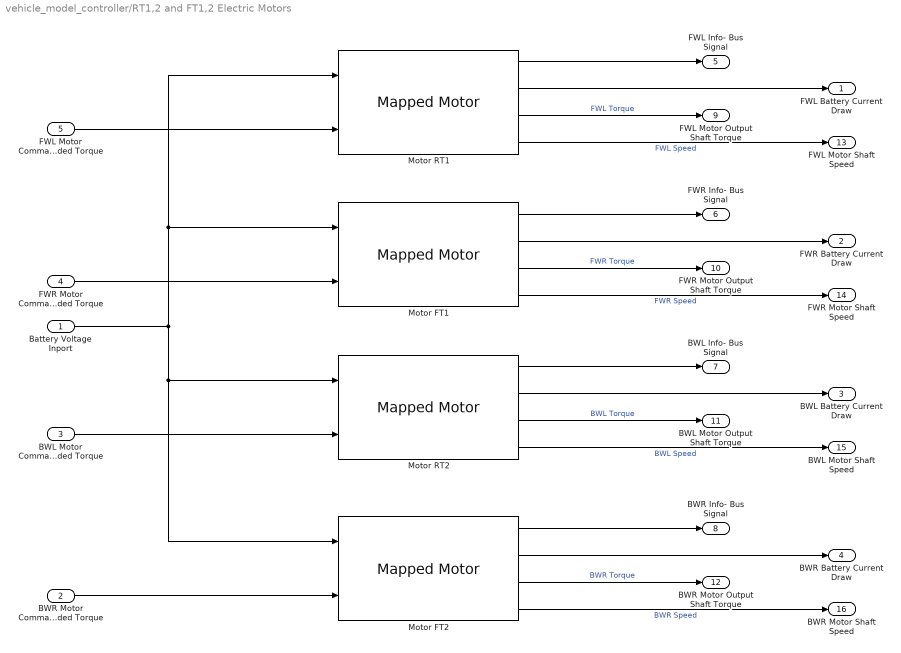
== system vehicle_model_controller/RT1,2 and FT1,2 Electric Motors ==
  Battery Voltage Inport : Inport
  BWR Motor Commanded Torque : Inport  Port=2
  BWL Motor Commanded Torque : Inport  Port=3
  "FWR Motor Commanded Torque " : Inport  Port=4
  FWL Motor Commanded Torque : Inport  Port=5
  Motor FT1 : autolibmappedmotor/Mapped Motor  port_config=Torque  param_by=Tabulated torque-speed envelope  w_t=[ 0 375 750 800 ]  T_t=[0.09 0.08 0.07 0]  torque_max=.1  power_max=30  Tc=0.02  param_loss=Single efficiency measurement  eff=100  w_eff=375  T_eff=0.08  Piron=0  Pbase=0  w_eff_bp=[-8000 -4000 0 4000 8000]  T_eff_bp=[0 0.03 0.06 0.09]  Temp_eff_bp=[233.15 293.15 373.15]  losses_table=[1.49 1.67 2.21 3.10; 0.42 0.69 1.14 2.03; 0.06 0.24 0.78 1.68; 0.42 0.69 1.14 2.03; 1.49 1.67 2.21 3.10]  losses_table_3d=cat(3,1.05*[1.49 1.67 2.21 3.10; 0.42 0.69 1.14 2.03; 0.06 0.24 0.78 1.68; 0.42 0.69 1.14 2.03; 1.49 1.67 2.21 3.10],[1.49 1.67 2.21 3.10; 0.42 0.69 1.14 2.03; 0.06 0.24 0.78 1.68; 0.42 0.69 1.14 2.03; 1.49 1.67 2.21 3.10],1.03*[1.49 1.67 2.21 3.10; 0.42 0.69 1.14 2.03; 0.06 0.24 0.78 1.68; 0.42 0.69 1.14 2.03; 1.49 1.67 2.21 3.10])  efficiency_table=[95 95 95 95; 95 95 95 95; 95 95 95 95; 95 95 95 95; 95 95 95 95]  efficiency_table_3d=cat(3,90*ones(5,4),95*ones(5,4),92*ones(5,4))  J=5e-6  b=1e-5  omega_o=0  T_t_extended=[0 0.07 0.08 0.09 0.08 0.07 0]  w_t_extended=[-800 -750 -375 0 375 750 800]  KLossIron=0  KLossCopper=0  x_w_eff_vec=[-8000 -4000 0 4000 8000]  x_T_eff_vec=[-0.09 -0.06 -0.03 0 0.03 0.06 0.09]  x_tmp_eff_vec=[233.15 293.15 373.15]  x_losses_mat=[3.1 2.21 1.67 1.49 1.67 2.21 3.1;2.03 1.14 0.69 0.42 0.69 1.14 2.03;1.68 0.78 0.24 0.06 0.24 0.78 1.68;2.03 1.14 0.69 0.42 0.69 1.14 2.03;3.1 2.21 1.67 1.49 1.67 2.21 3.1]  x_losses_mat_3d=cat(3,[3.255 2.3205 1.7535 1.5645 1.7535 2.3205 3.255;2.1315 1.197 0.7245 0.441 0.7245 1.197 2.1315;1.764 0.819 0.252 0.063 0.252 0.819 1.764;2.1315 1.197 0.7245 0.441 0.7245 1.197 2.1315;3.255 2.3205 1.7535 1.5645 1.7535 2.3205 3.255],[3.1 2.21 1.67 1.49 1.67 2.21 3.1;2.03 1.14 0.69 0.42 0.69 1.14 2.03;1.68 0.78 0.24 0.06 0.24 0.78 1.68;2.03 1.14 0.69 0.42 0.69 1.14 2.03;3.1 2.21 1.67 1.49 1.67 2.21 3.1],[3.193 2.2763 1.7201 1.5347 1.7201 2.2763 3.193;2.0909 1.1742 0.7107 0.4326 0.7107 1.1742 2.0909;1.7304 0.8034 0.2472 0.0618 0.2472 0.8034 1.7304;2.0909 1.1742 0.7107 0.4326 0.7107 1.1742 2.0909;3.193 2.2763 1.7201 1.5347 1.7201 2.2763 3.193])  CalLossMapData={}  CalLossWithTempMapData={}  aMode=1  RefBlkName='autolibmappedmotor/Mapped Motor'
      settings: SourceProductBaseCode=PW,MT,UV,VE,VP
  Motor FT2 : autolibmappedmotor/Mapped Motor  port_config=Torque  param_by=Tabulated torque-speed envelope  w_t=[ 0 375 750 800 ]  T_t=[0.09 0.08 0.07 0]  torque_max=.1  power_max=30  Tc=0.02  param_loss=Single efficiency measurement  eff=100  w_eff=375  T_eff=0.08  Piron=0  Pbase=0  w_eff_bp=[-8000 -4000 0 4000 8000]  T_eff_bp=[0 0.03 0.06 0.09]  Temp_eff_bp=[233.15 293.15 373.15]  losses_table=[1.49 1.67 2.21 3.10; 0.42 0.69 1.14 2.03; 0.06 0.24 0.78 1.68; 0.42 0.69 1.14 2.03; 1.49 1.67 2.21 3.10]  losses_table_3d=cat(3,1.05*[1.49 1.67 2.21 3.10; 0.42 0.69 1.14 2.03; 0.06 0.24 0.78 1.68; 0.42 0.69 1.14 2.03; 1.49 1.67 2.21 3.10],[1.49 1.67 2.21 3.10; 0.42 0.69 1.14 2.03; 0.06 0.24 0.78 1.68; 0.42 0.69 1.14 2.03; 1.49 1.67 2.21 3.10],1.03*[1.49 1.67 2.21 3.10; 0.42 0.69 1.14 2.03; 0.06 0.24 0.78 1.68; 0.42 0.69 1.14 2.03; 1.49 1.67 2.21 3.10])  efficiency_table=[95 95 95 95; 95 95 95 95; 95 95 95 95; 95 95 95 95; 95 95 95 95]  efficiency_table_3d=cat(3,90*ones(5,4),95*ones(5,4),92*ones(5,4))  J=5e-6  b=1e-5  omega_o=0  T_t_extended=[0 0.07 0.08 0.09 0.08 0.07 0]  w_t_extended=[-800 -750 -375 0 375 750 800]  KLossIron=0  KLossCopper=0  x_w_eff_vec=[-8000 -4000 0 4000 8000]  x_T_eff_vec=[-0.09 -0.06 -0.03 0 0.03 0.06 0.09]  x_tmp_eff_vec=[233.15 293.15 373.15]  x_losses_mat=[3.1 2.21 1.67 1.49 1.67 2.21 3.1;2.03 1.14 0.69 0.42 0.69 1.14 2.03;1.68 0.78 0.24 0.06 0.24 0.78 1.68;2.03 1.14 0.69 0.42 0.69 1.14 2.03;3.1 2.21 1.67 1.49 1.67 2.21 3.1]  x_losses_mat_3d=cat(3,[3.255 2.3205 1.7535 1.5645 1.7535 2.3205 3.255;2.1315 1.197 0.7245 0.441 0.7245 1.197 2.1315;1.764 0.819 0.252 0.063 0.252 0.819 1.764;2.1315 1.197 0.7245 0.441 0.7245 1.197 2.1315;3.255 2.3205 1.7535 1.5645 1.7535 2.3205 3.255],[3.1 2.21 1.67 1.49 1.67 2.21 3.1;2.03 1.14 0.69 0.42 0.69 1.14 2.03;1.68 0.78 0.24 0.06 0.24 0.78 1.68;2.03 1.14 0.69 0.42 0.69 1.14 2.03;3.1 2.21 1.67 1.49 1.67 2.21 3.1],[3.193 2.2763 1.7201 1.5347 1.7201 2.2763 3.193;2.0909 1.1742 0.7107 0.4326 0.7107 1.1742 2.0909;1.7304 0.8034 0.2472 0.0618 0.2472 0.8034 1.7304;2.0909 1.1742 0.7107 0.4326 0.7107 1.1742 2.0909;3.193 2.2763 1.7201 1.5347 1.7201 2.2763 3.193])  CalLossMapData={}  CalLossWithTempMapData={}  aMode=1  RefBlkName='autolibmappedmotor/Mapped Motor'
      settings: SourceProductBaseCode=PW,MT,UV,VE,VP
  Motor RT1 : autolibmappedmotor/Mapped Motor  port_config=Torque  param_by=Tabulated torque-speed envelope  w_t=[ 0 375 750 800 ]  T_t=[0.09 0.08 0.07 0]  torque_max=.1  power_max=30  Tc=0.02  param_loss=Single efficiency measurement  eff=100  w_eff=375  T_eff=0.08  Piron=0  Pbase=0  w_eff_bp=[-8000 -4000 0 4000 8000]  T_eff_bp=[0 0.03 0.06 0.09]  Temp_eff_bp=[233.15 293.15 373.15]  losses_table=[1.49 1.67 2.21 3.10; 0.42 0.69 1.14 2.03; 0.06 0.24 0.78 1.68; 0.42 0.69 1.14 2.03; 1.49 1.67 2.21 3.10]  losses_table_3d=cat(3,1.05*[1.49 1.67 2.21 3.10; 0.42 0.69 1.14 2.03; 0.06 0.24 0.78 1.68; 0.42 0.69 1.14 2.03; 1.49 1.67 2.21 3.10],[1.49 1.67 2.21 3.10; 0.42 0.69 1.14 2.03; 0.06 0.24 0.78 1.68; 0.42 0.69 1.14 2.03; 1.49 1.67 2.21 3.10],1.03*[1.49 1.67 2.21 3.10; 0.42 0.69 1.14 2.03; 0.06 0.24 0.78 1.68; 0.42 0.69 1.14 2.03; 1.49 1.67 2.21 3.10])  efficiency_table=[95 95 95 95; 95 95 95 95; 95 95 95 95; 95 95 95 95; 95 95 95 95]  efficiency_table_3d=cat(3,90*ones(5,4),95*ones(5,4),92*ones(5,4))  J=5e-6  b=1e-5  omega_o=0  T_t_extended=[0 0.07 0.08 0.09 0.08 0.07 0]  w_t_extended=[-800 -750 -375 0 375 750 800]  KLossIron=0  KLossCopper=0  x_w_eff_vec=[-8000 -4000 0 4000 8000]  x_T_eff_vec=[-0.09 -0.06 -0.03 0 0.03 0.06 0.09]  x_tmp_eff_vec=[233.15 293.15 373.15]  x_losses_mat=[3.1 2.21 1.67 1.49 1.67 2.21 3.1;2.03 1.14 0.69 0.42 0.69 1.14 2.03;1.68 0.78 0.24 0.06 0.24 0.78 1.68;2.03 1.14 0.69 0.42 0.69 1.14 2.03;3.1 2.21 1.67 1.49 1.67 2.21 3.1]  x_losses_mat_3d=cat(3,[3.255 2.3205 1.7535 1.5645 1.7535 2.3205 3.255;2.1315 1.197 0.7245 0.441 0.7245 1.197 2.1315;1.764 0.819 0.252 0.063 0.252 0.819 1.764;2.1315 1.197 0.7245 0.441 0.7245 1.197 2.1315;3.255 2.3205 1.7535 1.5645 1.7535 2.3205 3.255],[3.1 2.21 1.67 1.49 1.67 2.21 3.1;2.03 1.14 0.69 0.42 0.69 1.14 2.03;1.68 0.78 0.24 0.06 0.24 0.78 1.68;2.03 1.14 0.69 0.42 0.69 1.14 2.03;3.1 2.21 1.67 1.49 1.67 2.21 3.1],[3.193 2.2763 1.7201 1.5347 1.7201 2.2763 3.193;2.0909 1.1742 0.7107 0.4326 0.7107 1.1742 2.0909;1.7304 0.8034 0.2472 0.0618 0.2472 0.8034 1.7304;2.0909 1.1742 0.7107 0.4326 0.7107 1.1742 2.0909;3.193 2.2763 1.7201 1.5347 1.7201 2.2763 3.193])  CalLossMapData={}  CalLossWithTempMapData={}  aMode=1  RefBlkName='autolibmappedmotor/Mapped Motor'
      settings: SourceProductBaseCode=PW,MT,UV,VE,VP
  Motor RT2 : autolibmappedmotor/Mapped Motor  port_config=Torque  param_by=Tabulated torque-speed envelope  w_t=[ 0 375 750 800 ]  T_t=[0.09 0.08 0.07 0]  torque_max=.1  power_max=30  Tc=0.02  param_loss=Single efficiency measurement  eff=100  w_eff=375  T_eff=0.08  Piron=0  Pbase=0  w_eff_bp=[-8000 -4000 0 4000 8000]  T_eff_bp=[0 0.03 0.06 0.09]  Temp_eff_bp=[233.15 293.15 373.15]  losses_table=[1.49 1.67 2.21 3.10; 0.42 0.69 1.14 2.03; 0.06 0.24 0.78 1.68; 0.42 0.69 1.14 2.03; 1.49 1.67 2.21 3.10]  losses_table_3d=cat(3,1.05*[1.49 1.67 2.21 3.10; 0.42 0.69 1.14 2.03; 0.06 0.24 0.78 1.68; 0.42 0.69 1.14 2.03; 1.49 1.67 2.21 3.10],[1.49 1.67 2.21 3.10; 0.42 0.69 1.14 2.03; 0.06 0.24 0.78 1.68; 0.42 0.69 1.14 2.03; 1.49 1.67 2.21 3.10],1.03*[1.49 1.67 2.21 3.10; 0.42 0.69 1.14 2.03; 0.06 0.24 0.78 1.68; 0.42 0.69 1.14 2.03; 1.49 1.67 2.21 3.10])  efficiency_table=[95 95 95 95; 95 95 95 95; 95 95 95 95; 95 95 95 95; 95 95 95 95]  efficiency_table_3d=cat(3,90*ones(5,4),95*ones(5,4),92*ones(5,4))  J=5e-6  b=1e-5  omega_o=0  T_t_extended=[0 0.07 0.08 0.09 0.08 0.07 0]  w_t_extended=[-800 -750 -375 0 375 750 800]  KLossIron=0  KLossCopper=0  x_w_eff_vec=[-8000 -4000 0 4000 8000]  x_T_eff_vec=[-0.09 -0.06 -0.03 0 0.03 0.06 0.09]  x_tmp_eff_vec=[233.15 293.15 373.15]  x_losses_mat=[3.1 2.21 1.67 1.49 1.67 2.21 3.1;2.03 1.14 0.69 0.42 0.69 1.14 2.03;1.68 0.78 0.24 0.06 0.24 0.78 1.68;2.03 1.14 0.69 0.42 0.69 1.14 2.03;3.1 2.21 1.67 1.49 1.67 2.21 3.1]  x_losses_mat_3d=cat(3,[3.255 2.3205 1.7535 1.5645 1.7535 2.3205 3.255;2.1315 1.197 0.7245 0.441 0.7245 1.197 2.1315;1.764 0.819 0.252 0.063 0.252 0.819 1.764;2.1315 1.197 0.7245 0.441 0.7245 1.197 2.1315;3.255 2.3205 1.7535 1.5645 1.7535 2.3205 3.255],[3.1 2.21 1.67 1.49 1.67 2.21 3.1;2.03 1.14 0.69 0.42 0.69 1.14 2.03;1.68 0.78 0.24 0.06 0.24 0.78 1.68;2.03 1.14 0.69 0.42 0.69 1.14 2.03;3.1 2.21 1.67 1.49 1.67 2.21 3.1],[3.193 2.2763 1.7201 1.5347 1.7201 2.2763 3.193;2.0909 1.1742 0.7107 0.4326 0.7107 1.1742 2.0909;1.7304 0.8034 0.2472 0.0618 0.2472 0.8034 1.7304;2.0909 1.1742 0.7107 0.4326 0.7107 1.1742 2.0909;3.193 2.2763 1.7201 1.5347 1.7201 2.2763 3.193])  CalLossMapData={}  CalLossWithTempMapData={}  aMode=1  RefBlkName='autolibmappedmotor/Mapped Motor'
      settings: SourceProductBaseCode=PW,MT,UV,VE,VP
  FWL Battery Current Draw : Outport
  FWR Battery Current Draw : Outport  Port=2
  BWL Battery Current Draw : Outport  Port=3
  BWR Battery Current Draw : Outport  Port=4
  FWL Info- Bus Signal : Outport  Port=5
  FWR Info- Bus Signal : Outport  Port=6
  BWL Info- Bus Signal : Outport  Port=7
  BWR Info- Bus Signal : Outport  Port=8
  FWL Motor Output Shaft Torque : Outport  Port=9
  FWR Motor Output Shaft Torque : Outport  Port=10
  BWL Motor Output Shaft Torque : Outport  Port=11
  BWR Motor Output Shaft Torque : Outport  Port=12
  FWL Motor Shaft Speed : Outport  Port=13
  FWR Motor Shaft Speed : Outport  Port=14
  BWL Motor Shaft Speed : Outport  Port=15
  BWR Motor Shaft Speed : Outport  Port=16
  wires:
  Motor FT2/3 -> BWR Motor Output Shaft Torque/1  "BWR Torque"
  Battery Voltage Inport/1 -> Motor RT2/1, Motor FT2/1, Motor FT1/1, Motor RT1/1
  Motor RT1/1 -> FWL Info- Bus Signal/1
  FWL Motor Commanded Torque/1 -> Motor RT1/2
  "FWR Motor Commanded Torque "/1 -> Motor FT1/2
  Motor RT2/1 -> BWL Info- Bus Signal/1
  Motor FT1/1 -> FWR Info- Bus Signal/1
  Motor FT2/1 -> BWR Info- Bus Signal/1
  Motor FT1/4 -> FWR Motor Shaft Speed/1  "FWR Speed"
  BWR Motor Commanded Torque/1 -> Motor FT2/2
  Motor RT2/4 -> BWL Motor Shaft Speed/1  "BWL Speed"
  Motor RT2/2 -> BWL Battery Current Draw/1
  Motor FT2/4 -> BWR Motor Shaft Speed/1  "BWR Speed"
  Motor FT2/2 -> BWR Battery Current Draw/1
  Motor RT1/3 -> FWL Motor Output Shaft Torque/1  "FWL Torque"
  BWL Motor Commanded Torque/1 -> Motor RT2/2
  Motor RT1/4 -> FWL Motor Shaft Speed/1  "FWL Speed"
  Motor FT1/3 -> FWR Motor Output Shaft Torque/1  "FWR Torque"
  Motor RT2/3 -> BWL Motor Output Shaft Torque/1  "BWL Torque"
  Motor RT1/2 -> FWL Battery Current Draw/1
  Motor FT1/2 -> FWR Battery Current Draw/1

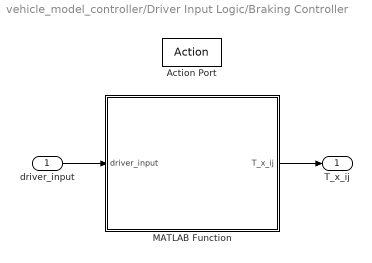
== system vehicle_model_controller/Driver Input Logic/Braking Controller ==
  driver_input : Inport
  Action Port : ActionPort  InitializeStates=reset  PropagateVarSize=During execution  ActionPortLabel=if(u1 <= 0)
  MATLAB Function : MATLAB Function  TreatAsAtomicUnit=on
  T_x_ij : Outport
  wires:
  driver_input/1 -> MATLAB Function/1(driver_input)
  MATLAB Function/1(T_x_ij) -> T_x_ij/1

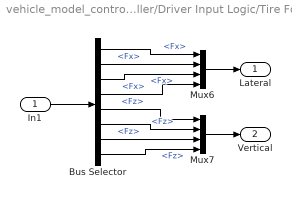
== system vehicle_model_controller/Driver Input Logic/Tire Force ==
  In1 : Inport
  Bus Selector : BusSelector  OutputSignals=BdyFrm.Forces.RearAxl.Rght.Fx,BdyFrm.Forces.RearAxl.Lft.Fx,BdyFrm.Forces.FrntAxl.Rght.Fx,BdyFrm.Forces.FrntAxl.Lft.Fx,BdyFrm.Forces.RearAxl.Rght.Fz,BdyFrm.Forces.RearAxl.Lft.Fz,BdyFrm.Forces.FrntAxl.Rght.Fz,BdyFrm.Forces.FrntAxl.Lft.Fz
  Mux6 : Mux
  Mux7 : Mux
  Lateral : Outport
  Vertical : Outport  Port=2
  wires:
  Bus Selector/2 -> Mux6/2  "<Fx>"
  Bus Selector/8 -> Mux7/4  "<Fz>"
  Bus Selector/5 -> Mux7/1  "<Fz>"
  Bus Selector/6 -> Mux7/2  "<Fz>"
  Bus Selector/1 -> Mux6/1  "<Fx>"
  Mux6/1 -> Lateral/1
  Bus Selector/4 -> Mux6/4  "<Fx>"
  Bus Selector/3 -> Mux6/3  "<Fx>"
  Bus Selector/7 -> Mux7/3  "<Fz>"
  Mux7/1 -> Vertical/1
  In1/1 -> Bus Selector/1

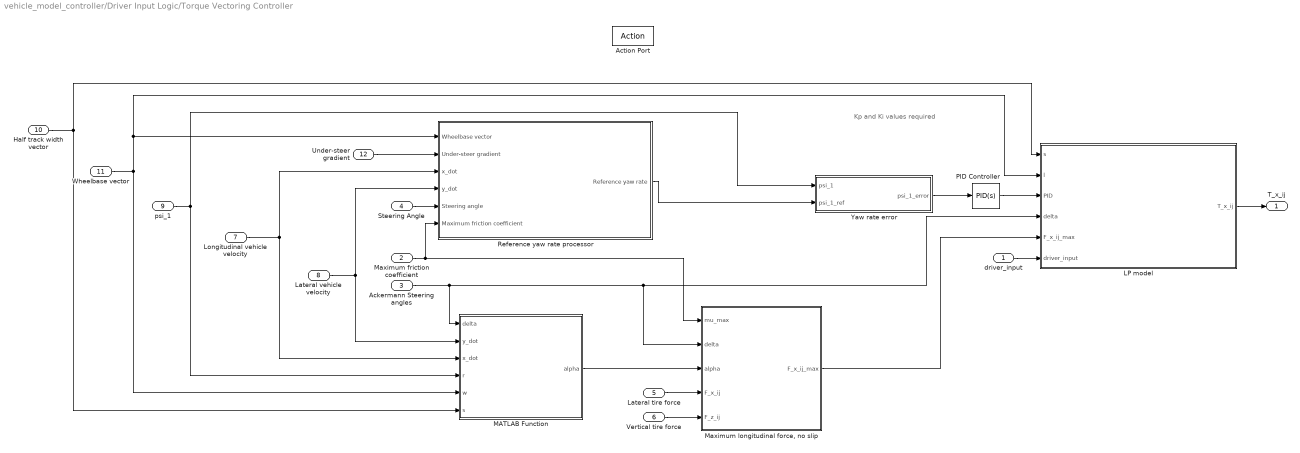
== system vehicle_model_controller/Driver Input Logic/Torque Vectoring Controller ==
  note: Kp and Ki values required
  driver_input : Inport
  Maximum friction coefficient : Inport  Port=2
  "Ackermann Steering angles " : Inport  Port=3
  Steering Angle : Inport  Port=4
  Lateral tire force : Inport  Port=5
  Vertical tire force : Inport  Port=6
  Longitudinal vehicle velocity : Inport  Port=7
  Lateral vehicle velocity : Inport  Port=8
  psi_1 : Inport  Port=9
  Half track width vector : Inport  Port=10
  Wheelbase vector : Inport  Port=11
  Under-steer gradient : Inport  Port=12
  Action Port : ActionPort  InitializeStates=reset  PropagateVarSize=During execution  ActionPortLabel=else
  LP model : MATLAB Function  TreatAsAtomicUnit=on
  MATLAB Function : MATLAB Function  TreatAsAtomicUnit=on
  "Maximum longitudinal force, no slip" : MATLAB Function  TreatAsAtomicUnit=on
  PID Controller : pid_lib/PID Controller  Controller=PID  Form=Parallel  TimeDomain=Continuous-time  UseExternalTs=off  SampleTime=-1  IntegratorMethod=Forward Euler  FilterMethod=Forward Euler  ControllerParametersSource=internal  P=1  I=1  D=0  UseFilter=on  N=100  TunerSelectOption=Transfer Function Based (PID Tuner App)  InitialConditionSource=internal  InitialConditionForIntegrator=0  InitialConditionForFilter=0  DifferentiatorICPrevScaledInput=0  ExternalReset=none  TrackingMode=off  Kt=1  LimitOutput=off  SatLimitsSource=internal  UpperSaturationLimit=inf  LowerSaturationLimit=-inf  LinearizeAsGain=on  AntiWindupMode=none  Kb=1  POutMin=[]  POutMax=[]  IOutMin=[]  IOutMax=[]  DOutMin=[]  DOutMax=[]  NOutMin=[]  NOutMax=[]  SumOutMin=[]  SumOutMax=[]  SaturationOutMin=[]  SaturationOutMax=[]  PParamMin=[]  PParamMax=[]  IParamMin=[]  IParamMax=[]  DParamMin=[]  DParamMax=[]  NParamMin=[]  NParamMax=[]  KbParamMin=[]  KbParamMax=[]  KtParamMin=[]  KtParamMax=[]  KbOutMin=[]  KbOutMax=[]  KtOutMin=[]  KtOutMax=[]  IntegratorOutMin=[]  IntegratorOutMax=[]  FilterOutMin=[]  FilterOutMax=[]  SumI1OutMin=[]  SumI1OutMax=[]  SumI2OutMin=[]  SumI2OutMax=[]  SumI3OutMin=[]  SumI3OutMax=[]  SumI4OutMin=[]  SumI4OutMax=[]  SumDOutMin=[]  SumDOutMax=[]  DifferentiatorOutMin=[]  DifferentiatorOutMax=[]  FilterDiffOutCoefMin=[]  FilterDiffOutCoefMax=[]  ReciprocalOutMin=[]  ReciprocalOutMax=[]  SumDenOutMin=[]  SumDenOutMax=[]  SumNumOutMin=[]  SumNumOutMax=[]  DivideOutMin=[]  DivideOutMax=[]  UdiffTsProdOutMin=[]  UdiffTsProdOutMax=[]  NTsProdOutMin=[]  NTsProdOutMax=[]  UintegralTsProdOutMin=[]  UintegralTsProdOutMax=[]  UngainTsProdOutMin=[]  UngainTsProdOutMax=[]  IntegratorContinuousStateAttributes=''  IntegratorStateMustResolveToSignalObject=off  IntegratorRTWStateStorageClass=Auto  FilterContinuousStateAttributes=''  FilterStateMustResolveToSignalObject=off  FilterRTWStateStorageClass=Auto  ParallelPVariant=InternalParameters  IdealPVariant=Disabled  IVariant=InternalParameters  DVariant=InternalParameters  IntegratorVariant=Continuous  SatVariant=Disabled  AWVariant=Passthrough  PCopyVariant=Disabled  TRVariant=Disabled  FdbkBlocksVariant=Forward  IdealPFdbkVariant=Disabled  SatFdbkVariant=Disabled  DerivativeFilterVariant=ContFilter  NVariant=InternalParameters  NCopyVariant=Disabled  FilterICVariant=InternalICsFilter  IntegratorICVariant=InternalICs  ExternalResetVariant=Disabled  TRSumVariant=Passthrough  SumFdbkVariant=Disabled  SumVariant=Sum_PID  TsampFilterVariant=InternalTs  TsampNgainVariant=Passthrough  TsampIntegralVariant=Passthrough  ExternalSaturationOutDataTypeStr=Inherit: Same as second input
  Reference yaw rate processor : Subsystem
  Yaw rate error : MATLAB Function  TreatAsAtomicUnit=on
  T_x_ij : Outport
  wires:
  PID Controller/1 -> LP model/3(PID)
  Maximum friction coefficient/1 -> Reference yaw rate processor/6(Maximum friction coefficient), "Maximum longitudinal force, no slip"/1(mu_max)
  Under-steer gradient/1 -> Reference yaw rate processor/2(Under-steer gradient)
  Reference yaw rate processor/1(Reference yaw rate) -> Yaw rate error/2(psi_1_ref)
  Yaw rate error/1(psi_1_error) -> PID Controller/1
  Half track width vector/1 -> MATLAB Function/6(s), LP model/1(s)
  Wheelbase vector/1 -> Reference yaw rate processor/1(Wheelbase vector), LP model/2(l), MATLAB Function/5(w)
  psi_1/1 -> Yaw rate error/1(psi_1), MATLAB Function/4(r)
  "Maximum longitudinal force, no slip"/1(F_x_ij_max) -> LP model/5(F_x_ij_max)
  Lateral tire force/1 -> "Maximum longitudinal force, no slip"/4(F_x_ij)
  Vertical tire force/1 -> "Maximum longitudinal force, no slip"/5(F_z_ij)
  MATLAB Function/1(alpha) -> "Maximum longitudinal force, no slip"/3(alpha)
  Longitudinal vehicle velocity/1 -> Reference yaw rate processor/3(x_dot), MATLAB Function/3(x_dot)
  Lateral vehicle velocity/1 -> Reference yaw rate processor/4(y_dot), MATLAB Function/2(y_dot)
  LP model/1(T_x_ij) -> T_x_ij/1
  "Ackermann Steering angles "/1 -> "Maximum longitudinal force, no slip"/2(delta), LP model/4(delta), MATLAB Function/1(delta)
  driver_input/1 -> LP model/6(driver_input)
  Steering Angle/1 -> Reference yaw rate processor/5("Steering angle ")

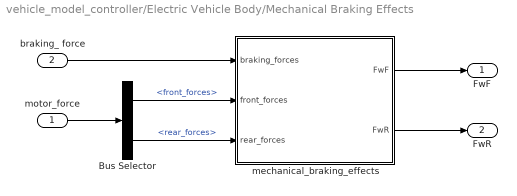
== system vehicle_model_controller/Electric Vehicle Body/Mechanical Braking Effects ==
  motor_force : Inport
  braking_	force : Inport  Port=2
  Bus Selector : BusSelector  OutputSignals=front_forces,rear_forces
  mechanical_braking_effects : MATLAB Function  TreatAsAtomicUnit=on
  FwF : Outport
  FwR : Outport  Port=2
  wires:
  mechanical_braking_effects/1(FwF) -> FwF/1
  braking_	force/1 -> mechanical_braking_effects/1(braking_forces)
  mechanical_braking_effects/2(FwR) -> FwR/1
  Bus Selector/1 -> mechanical_braking_effects/2(front_forces)  "<front_forces>"
  Bus Selector/2 -> mechanical_braking_effects/3(rear_forces)  "<rear_forces>"
  motor_force/1 -> Bus Selector/1
